simulink model "simulation"  (R2023a)
settings: Solver=FixedStepAuto  StartTime=0.0  StopTime=10  FixedStep=0.05  RelTol=1e-3
undefined symbols (not defined in the file): A_, B_, K, starting_position, target_position
settings Model: Creator=valer  LastModifiedBy=valer

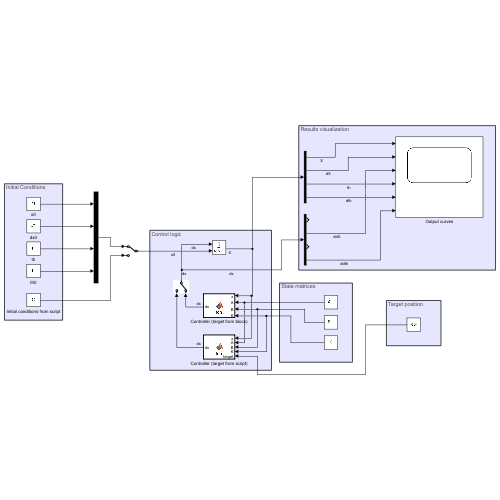
[thumbnail: Simulink's stored preview of the top-level diagram]
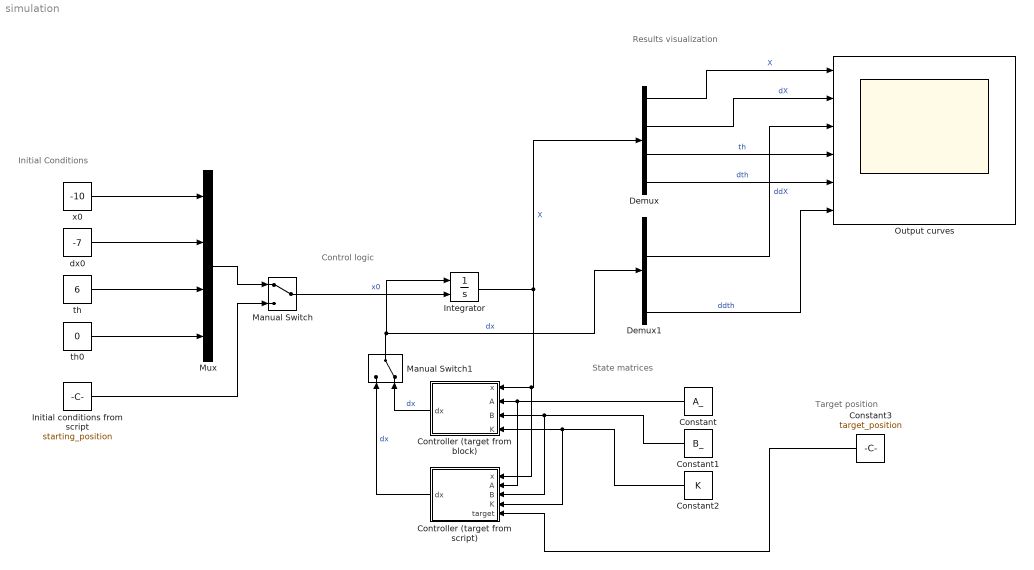
== system simulation ==
  note: Target position
  note: State matrices
  note: Initial Conditions
  note: Control logic
  note: Results visualization
  Constant : Constant  Value=A_
  Constant1 : Constant  Value=B_
  Constant2 : Constant  Value=K
  Constant3 : Constant  Value=target_position
  Controller (target from block) : MATLAB Function  TreatAsAtomicUnit=on
  Controller (target from script) : MATLAB Function  TreatAsAtomicUnit=on
  Demux : Demux
  Demux1 : Demux
  Initial conditions from script : Constant  Value=starting_position
  Integrator : Integrator  InitialConditionSource=external  InitialCondition=[0 0 15 0]'
  Manual Switch : ManualSwitch
  Manual Switch1 : ManualSwitch  CurrentSetting=0
  Mux : Mux
  Output curves : Scope  NumInputPorts=6
  dx0 : Constant  Value=-7
  th : Constant  Value=6
  th0 : Constant  Value=0
  x0 : Constant  Value=-10
  wires:
  Constant1/1 -> Controller (target from script)/3(B), Controller (target from block)/3(B)
  Demux/4 -> Output curves/5  "dth"
  Demux/1 -> Output curves/1  "X"
  Demux1/2 -> Output curves/3  "ddX"
  x0/1 -> Mux/1
  th/1 -> Mux/3
  th0/1 -> Mux/4
  dx0/1 -> Mux/2
  Mux/1 -> Manual Switch/1
  Integrator/1 -> Controller (target from script)/1(x), Controller (target from block)/1(x), Demux/1  "X"
  Demux/2 -> Output curves/2  "dX"
  Constant2/1 -> Controller (target from script)/4(K), Controller (target from block)/4(K)
  Demux1/4 -> Output curves/6  "ddth"
  Demux/3 -> Output curves/4  "th"
  Constant/1 -> Controller (target from script)/2(A), Controller (target from block)/2(A)
  Manual Switch1/1 -> Integrator/1, Demux1/1  "dx"
  Manual Switch/1 -> Integrator/2  "x0"
  Initial conditions from script/1 -> Manual Switch/2
  Controller (target from block)/1(dx) -> Manual Switch1/2  "dx"
  Controller (target from script)/1(dx) -> Manual Switch1/1  "dx"
  Constant3/1 -> Controller (target from script)/5(target)

== matlab function simulation/Controller (target from script) ==
  data: x input; dx output; A input; B input; K input; target input
function dx = fcn(x,A,B,K,target)
    % Allows for the definition of the target position inside of the script
    % at the expanse of less freedom in the choices
    dx = A*x + B * (-K' * (x - target));

== matlab function simulation/Controller (target from block) ==
  data: x input; dx output; A input; B input; K input
function dx = fcn(x,A,B,K)
    % Select the target state (X dX th dth) through this variable
    target = [0 0 0 0]'; % Free states can be written as [x(1) ... x(4)]
    dx = A*x + B * (-K' * (x - target));
